simulink subsystem "InjectorNHNE"  (R2020b)
settings: Solver=VariableStepAuto  StartTime=0.0  StopTime=10.0  RelTol=1e-3
model mask{dischargeCoeff=0.8, numHolesPort1=5, numHolesPort2=5, holeAreaPort1=2e-5, holeAreaPort2=2e-5}
  mask prompts: dischargeCoeff "Cd"; numHolesPort1 "Number of holes port 1"; numHolesPort2 "Number of holes port 2"; holeAreaPort1 "Single hole area port 1 (m^2)"; holeAreaPort2 "Single hole area port 2 (m^2)"
libraries: nesl_utility x6, fl_lib x3, SimscapeCustomBlocks_lib x2
settings Model: Creator=Edward  LastModifiedBy=Edward

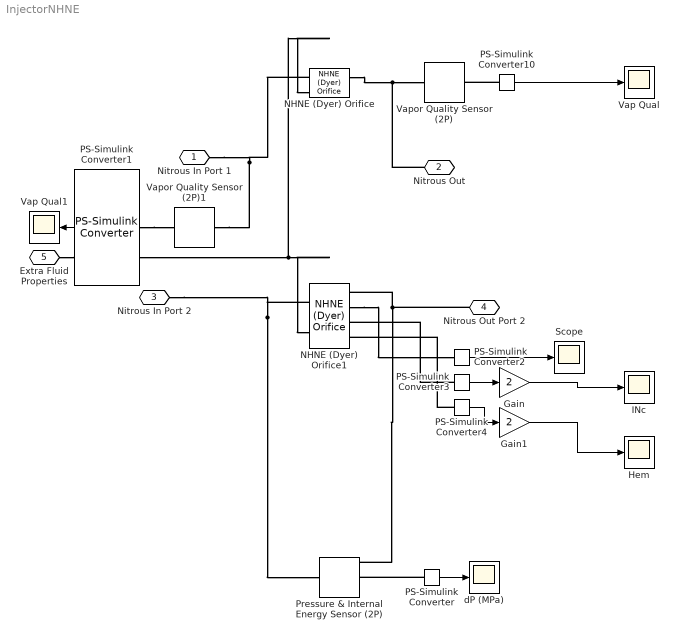
== system InjectorNHNE ==
  Gain : Gain  Gain=2
  Gain1 : Gain  Gain=2
  Hem : Scope
  INc : Scope
  NHNE (Dyer) Orifice : SimscapeCustomBlocks_lib/NHNE (Dyer) Orifice  area=Sim.preInjectorPipe.crossSection m^2  orifice_area=numHolesPort1 * holeAreaPort1 m^2  Cd=dischargeCoeff
      settings: InternalSimscapePortConfiguration="{\"Bottom\":[],\"Left\":[{\"id\":\"A\",\"label\":\"A\",\"type\":\"foundation.two_phase_fluid.two_phase_fluid\"}],\"Right\":[{\"id\":\"B\",\"label\":\"B\",\"type\":\"foundation.two_phase_fluid.two_phase_fluid\"},{\"id\":\"kOut\",\"label\":\"K\",\"type\":\"output\"},{\"id\":\"MInc\",\"label\":\"MInc\",\"type\":\"output\"},{\"id\":\"MHEM\",\"label\":\"MHEM\",\"type\":\"output\"}],\"Top\":[{\"id\":\"Props\",\"label\":\"Props\",\"type\":\"SimscapeCustomBlocks.customFluidDomain.extra_two_phase_fluid_props\"}]}"
  NHNE (Dyer) Orifice1 : SimscapeCustomBlocks_lib/NHNE (Dyer) Orifice  area=Sim.preInjectorPipe.crossSection m^2  orifice_area=numHolesPort2 * holeAreaPort2 m^2  Cd=dischargeCoeff
      settings: InternalSimscapePortConfiguration="{\"Bottom\":[],\"Left\":[{\"id\":\"A\",\"label\":\"A\",\"type\":\"foundation.two_phase_fluid.two_phase_fluid\"}],\"Right\":[{\"id\":\"B\",\"label\":\"B\",\"type\":\"foundation.two_phase_fluid.two_phase_fluid\"},{\"id\":\"kOut\",\"label\":\"K\",\"type\":\"output\"},{\"id\":\"MInc\",\"label\":\"MInc\",\"type\":\"output\"},{\"id\":\"MHEM\",\"label\":\"MHEM\",\"type\":\"output\"}],\"Top\":[{\"id\":\"Props\",\"label\":\"Props\",\"type\":\"SimscapeCustomBlocks.customFluidDomain.extra_two_phase_fluid_props\"}]}"
  PS-Simulink Converter{,1..4,10} (6 alike) : nesl_utility/PS-Simulink Converter  PhysicalDomain=network_engine_domain  SubClassName=ps_output  LeftPortType=input  RightPortType=output  PseudoPeriodic=off  Frequencies=[]  Unit=inherit  AffineConversion=off
  Pressure & Internal Energy Sensor (2P) : fl_lib/Two-Phase Fluid/Sensors/Pressure & Internal Energy Sensor (2P)
      settings: SourceProductBaseCode=SS  InternalSimscapePortConfiguration="{\"Bottom\":[],\"Left\":[{\"id\":\"A\",\"label\":\"A\",\"type\":\"foundation.two_phase_fluid.two_phase_fluid\"}],\"Right\":[{\"id\":\"B\",\"label\":\"B\",\"type\":\"foundation.two_phase_fluid.two_phase_fluid\"},{\"id\":\"P\",\"label\":\"P\",\"type\":\"output\"},{\"id\":\"U\",\"label\":\"U\",\"type\":\"output\"}],\"Top\":[]}"
  Scope : Scope
  Vap Qual : Scope
  Vap Qual1 : Scope
  Vapor Quality Sensor (2P) : fl_lib/Two-Phase Fluid/Sensors/Vapor Quality Sensor (2P)  vapor_fraction_spec=foundation.enum.vapor_fraction_spec.quality
      settings: SourceProductBaseCode=SS  InternalSimscapePortConfiguration="{\"Bottom\":[],\"Left\":[{\"id\":\"A\",\"label\":\"A\",\"type\":\"foundation.two_phase_fluid.two_phase_fluid\"}],\"Right\":[{\"id\":\"X\",\"label\":\"X\",\"type\":\"output\"}],\"Top\":[]}"
  Vapor Quality Sensor (2P)1 : fl_lib/Two-Phase Fluid/Sensors/Vapor Quality Sensor (2P)  vapor_fraction_spec=foundation.enum.vapor_fraction_spec.quality
      settings: SourceProductBaseCode=SS  InternalSimscapePortConfiguration="{\"Bottom\":[],\"Left\":[{\"id\":\"A\",\"label\":\"A\",\"type\":\"foundation.two_phase_fluid.two_phase_fluid\"}],\"Right\":[{\"id\":\"X\",\"label\":\"X\",\"type\":\"output\"}],\"Top\":[]}"
  dP (MPa) : Scope
  Nitrous In Port 1 : PMIOPort  Side=Left
  Nitrous Out : PMIOPort  Port=2  Side=Right
  Nitrous In Port 2 : PMIOPort  Port=3  Side=Left
  Nitrous Out Port 2 : PMIOPort  Port=4  Side=Right
  Extra Fluid Properties : PMIOPort  Port=5  Side=Left
  wires:
  PS-Simulink Converter1/1 -> Vap Qual1/1
  PS-Simulink Converter10/1 -> Vap Qual/1
  PS-Simulink Converter/1 -> dP (MPa)/1
  PS-Simulink Converter2/1 -> Scope/1
  PS-Simulink Converter3/1 -> Gain/1
  PS-Simulink Converter4/1 -> Gain1/1
  Gain/1 -> INc/1
  Gain1/1 -> Hem/1
  connections:
  Nitrous Out Port 2/RConn1 -- Pressure & Internal Energy Sensor (2P)/RConn1 -- NHNE (Dyer) Orifice1/RConn1
  Nitrous In Port 2/RConn1 -- Pressure & Internal Energy Sensor (2P)/LConn1 -- NHNE (Dyer) Orifice1/LConn1
  Vapor Quality Sensor (2P)1/LConn1 -- Nitrous In Port 1/RConn1 -- NHNE (Dyer) Orifice/LConn1
  Nitrous Out/RConn1 -- Vapor Quality Sensor (2P)/LConn1 -- NHNE (Dyer) Orifice/RConn1
  Extra Fluid Properties/RConn1 -- NHNE (Dyer) Orifice1/LConn2 -- NHNE (Dyer) Orifice/LConn2
  PS-Simulink Converter1/LConn1 -- Vapor Quality Sensor (2P)1/RConn1
  PS-Simulink Converter10/LConn1 -- Vapor Quality Sensor (2P)/RConn1
  PS-Simulink Converter/LConn1 -- Pressure & Internal Energy Sensor (2P)/RConn2
  NHNE (Dyer) Orifice1/RConn2 -- PS-Simulink Converter2/LConn1
  PS-Simulink Converter3/LConn1 -- NHNE (Dyer) Orifice1/RConn3
  PS-Simulink Converter4/LConn1 -- NHNE (Dyer) Orifice1/RConn4
